simulink model "sampleModel1557"  (R2023a)
settings: Solver=VariableStepAuto  StartTime=0.0  StopTime=10.0  RelTol=1e-3
libraries: hdlsllib x3, simulink x1
settings Model: Creator=user1  LastModifiedBy=user1

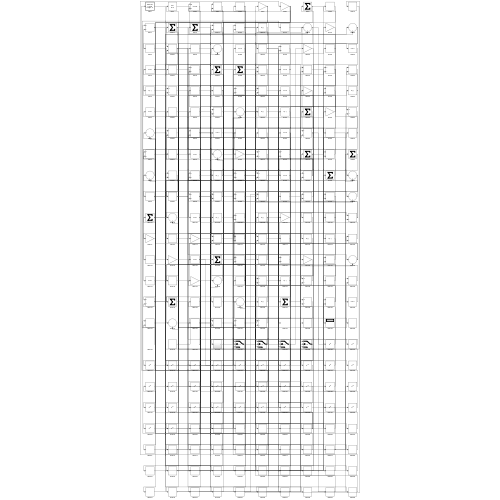
[thumbnail: Simulink's stored preview of the top-level diagram]
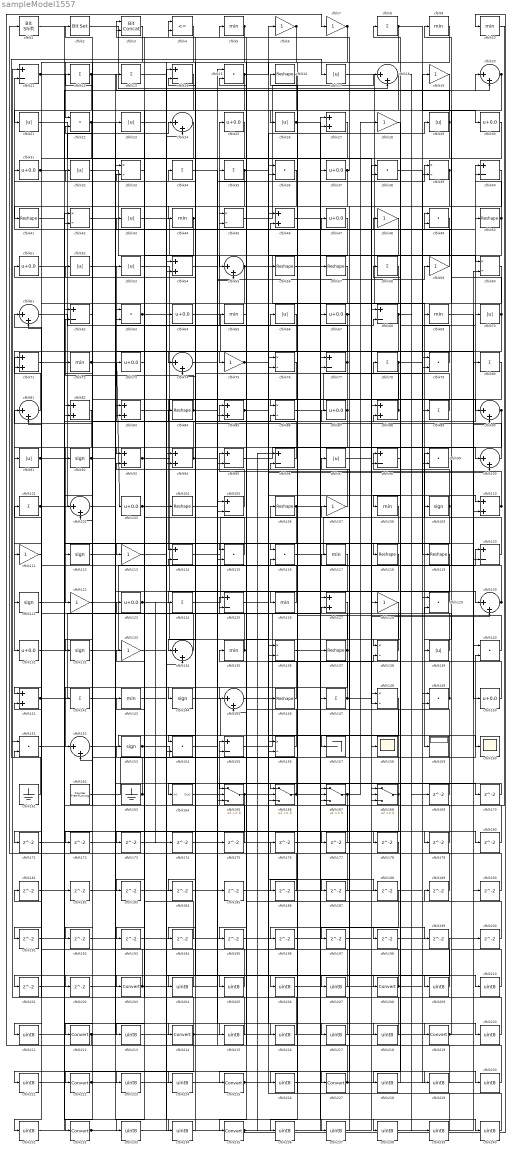
== system sampleModel1557 ==
  cfblk1 : hdlsllib/Logic and Bit Operations/Bit Shift  mode=Shift Left Logical  N=0
  cfblk{5,9..10,44,65,69,72,108,117,126,135,143} (12 alike) : MinMax
  cfblk{18,20,24,55,61,74,81,90,100,102,130,134,145,152} (14 alike) : Sum  Inputs=|++
  cfblk{8,12..13,34..35,58,78,80,89,101,124,142,147} (13 alike) : Sum  Inputs=+
  cfblk{25,30..31,37,47,51,64,67,73,87,103,123,131,150} (14 alike) : Bias  Bias=0.0  SaturateOnIntegerOverflow=off
  cfblk{16,41,50,56..57,84,104,106,118..119,137,146} (12 alike) : Reshape
  cfblk{11,14,40,62,68,77,95..96,98,105,114,120,125,155} (14 alike) : Sum  Inputs=+-
  cfblk{6..7,19,28,48,59,75,107,111,113,122,128,133} (13 alike) : Gain
  cfblk{92,109,112,121,132,144,153} (7 alike) : Signum
  cfblk{27,46,54,71,82..83,85,88,93..94,110,127,141} (13 alike) : Sum
  cfblk{15,22,36,38,49,63,79,99,115..116,129,140,149,151,154} (15 alike) : DotProduct  OutDataTypeStr=Inherit: Inherit via internal rule
  cfblk{33,39,42,45,60,76,86,136,138,148,156} (11 alike) : Product  Inputs=*/  RndMeth=Zero  SaturateOnIntegerOverflow=on
  cfblk{17,21,23,26,29,32,43,52..53,66,70,91,97,139} (14 alike) : Abs  SaturateOnIntegerOverflow=off
  cfblk157 : Terminator
  cfblk158 : Scope
  cfblk159 : Display
  cfblk160 : Scope
  cfblk161 : Ground
  cfblk162 : hdlsllib/Sources/Counter Free-Running  NumBits=16  tsamp=-1
  cfblk163 : Ground
  cfblk164 : Subsystem
      settings: LibrarySourceBlock=|
      | hdlsllib/Ports &
      | Subsystems/Subsystem
  cfblk{165..168} (4 alike) : Switch  SaturateOnIntegerOverflow=off  InputSameDT=off
  cfblk{169..202} (34 alike) : Delay  SampleTime=1
  cfblk2 : simulink/Logic and Bit Operations/Bit Set  iBit=0
      settings: LibrarySourceBlock=|
      | hdlsllib/Logic and Bit
      | Operations/Bit Set
  cfblk{203,208,212,214,219,222,225,227,232,235} (10 alike) : DataTypeConversion  SaturateOnIntegerOverflow=off  RndMeth=Floor
  cfblk{204..207,209..211,213,215..218,220..221,223..224,226,228..231,233..234,236..240} (28 alike) : DataTypeConversion  OutDataTypeStr=uint8  SaturateOnIntegerOverflow=off  RndMeth=Floor
  cfblk3 : hdlsllib/Logic and Bit Operations/Bit Concat  numInputs=2
  cfblk4 : RelationalOperator  Operator=<=  OutDataTypeStr=boolean  InputSameDT=off
  wires:
  cfblk14/1 -> cfblk232/1
  cfblk54/1 -> cfblk219/1
  cfblk67/1 -> cfblk95/2, cfblk85/2, cfblk187/1
  cfblk66/1 -> cfblk131/1
  cfblk53/1 -> cfblk126/1
  cfblk40/1 -> cfblk157/1
  cfblk19/1 -> cfblk225/1
  cfblk71/1 -> cfblk24/1
  cfblk123/1 -> cfblk146/1, cfblk174/1
  cfblk78/1 -> cfblk114/1, cfblk70/1
  cfblk95/1 -> cfblk100/1
  cfblk136/1 -> cfblk57/1
  cfblk37/1 -> cfblk4/1, cfblk44/1
  cfblk124/1 -> cfblk67/1
  cfblk146/1 -> cfblk135/1
  cfblk161/1 -> cfblk17/1
  cfblk85/1 -> cfblk145/2, cfblk188/1, cfblk220/1
  cfblk100/1 -> cfblk4/2
  cfblk111/1 -> cfblk141/1
  cfblk63/1 -> cfblk147/1, cfblk64/1
  cfblk147/1 -> cfblk16/1, cfblk130/2
  cfblk139/1 -> cfblk97/1
  cfblk87/1 -> cfblk86/1, cfblk136/2, cfblk173/1
  cfblk93/1 -> cfblk118/1, cfblk240/1
  cfblk98/1 -> cfblk8/1
  cfblk155/1 -> cfblk37/1
  cfblk156/1 -> cfblk5/1
  cfblk96/1 -> cfblk53/1
  cfblk17/1 -> cfblk159/1
  cfblk120/1 -> cfblk99/1
  cfblk56/1 -> cfblk110/1
  cfblk3/1 -> cfblk22/1
  cfblk16/1 -> cfblk113/1
  cfblk105/1 -> cfblk3/1
  cfblk112/1 -> cfblk130/1
  cfblk89/1 -> cfblk51/1
  cfblk10/1 -> cfblk155/1
  cfblk52/1 -> cfblk75/1
  cfblk9/1 -> cfblk144/1
  cfblk82/1 -> cfblk122/1
  cfblk166/1 -> cfblk32/1, cfblk81/1, cfblk120/1
  cfblk45/1 -> cfblk18/1
  cfblk114/1 -> cfblk77/2
  cfblk129/1 -> cfblk66/1
  cfblk162/1 -> cfblk140/2
  cfblk72/1 -> cfblk103/1, cfblk142/1
  cfblk61/1 -> cfblk68/2
  cfblk151/1 -> cfblk214/1
  cfblk39/1 -> cfblk171/1, cfblk228/1
  cfblk28/1 -> cfblk108/1
  cfblk118/1 -> cfblk165/1
  cfblk22/1 -> cfblk74/1, cfblk167/3, cfblk211/1
  cfblk141/1 -> cfblk56/1, cfblk180/1
  cfblk91/1 -> cfblk25/1, cfblk120/2
  cfblk2/1 -> cfblk18/2
  cfblk57/1 -> cfblk134/1
  cfblk33/1 -> cfblk203/1
  cfblk101/1 -> cfblk40/1, cfblk88/2
  cfblk55/1 -> cfblk60/1, cfblk99/2, cfblk91/1
  cfblk106/1 -> cfblk137/1, cfblk132/1
  cfblk165/1 -> cfblk138/2, cfblk223/1
  cfblk117/1 -> cfblk164/1(In1)
  cfblk25/1 -> cfblk154/1
  cfblk18/1 -> cfblk145/1, cfblk169/1
  cfblk50/1 -> cfblk40/2, cfblk148/2
  cfblk164/1(Out1) -> cfblk39/1
  cfblk21/1 -> cfblk128/1
  cfblk75/1 -> cfblk29/1, cfblk110/2
  cfblk20/1 -> cfblk69/1, cfblk26/1
  cfblk143/1 -> cfblk104/1
  cfblk79/1 -> cfblk58/1
  cfblk68/1 -> cfblk121/1, cfblk239/1
  cfblk15/1 -> cfblk6/1, cfblk152/2, cfblk100/2
  cfblk59/1 -> cfblk11/2
  cfblk130/1 -> cfblk49/1, cfblk74/2
  cfblk64/1 -> cfblk150/1
  cfblk153/1 -> cfblk155/2, cfblk116/2
  cfblk48/1 -> cfblk227/1
  cfblk7/1 -> cfblk124/1, cfblk21/1, cfblk186/1, cfblk204/1
  cfblk43/1 -> cfblk55/1
  cfblk32/1 -> cfblk79/2
  cfblk83/1 -> cfblk90/1
  cfblk133/1 -> cfblk208/1
  cfblk104/1 -> cfblk86/2
  cfblk144/1 -> cfblk167/1
  cfblk65/1 -> cfblk115/1
  cfblk167/1 -> cfblk28/1, cfblk195/1, cfblk197/1
  cfblk80/1 -> cfblk212/1
  cfblk148/1 -> cfblk156/2
  cfblk115/1 -> cfblk83/1
  cfblk74/1 -> cfblk47/1
  cfblk121/1 -> cfblk84/1
  cfblk84/1 -> cfblk62/2, cfblk49/2
  cfblk6/1 -> cfblk76/2, cfblk205/1
  cfblk132/1 -> cfblk114/2
  cfblk109/1 -> cfblk98/1, cfblk213/1
  cfblk73/1 -> cfblk93/1
  cfblk107/1 -> cfblk45/1
  cfblk138/1 -> cfblk101/1
  cfblk38/1 -> cfblk119/1
  cfblk4/1 -> cfblk41/1
  cfblk77/1 -> cfblk63/1, cfblk193/1
  cfblk24/1 -> cfblk82/2
  cfblk81/1 -> cfblk71/1
  cfblk149/1 -> cfblk125/1, cfblk85/1
  cfblk62/1 -> cfblk92/1
  cfblk69/1 -> cfblk90/2
  cfblk36/1 -> cfblk222/1
  cfblk168/1 -> cfblk117/1, cfblk226/1
  cfblk90/1 -> cfblk111/1, cfblk167/2
  cfblk102/1 -> cfblk50/1
  cfblk103/1 -> cfblk166/1, cfblk116/1
  cfblk163/1 -> cfblk83/2, cfblk72/1
  cfblk152/1 -> cfblk160/1
  cfblk70/1 -> cfblk9/1, cfblk194/1
  cfblk26/1 -> cfblk198/1, cfblk199/1
  cfblk122/1 -> cfblk89/1
  cfblk11/1 -> cfblk201/1, cfblk237/1
  cfblk47/1 -> cfblk166/2
  cfblk97/1 -> cfblk38/1
  cfblk60/1 -> cfblk102/1
  cfblk137/1 -> cfblk152/1, cfblk12/1
  cfblk140/1 -> cfblk106/1
  cfblk86/1 -> cfblk39/2
  cfblk76/1 -> cfblk105/2
  cfblk128/1 -> cfblk166/3
  cfblk150/1 -> cfblk107/1
  cfblk127/1 -> cfblk235/1
  cfblk12/1 -> cfblk73/1, cfblk81/2
  cfblk110/1 -> cfblk78/1, cfblk95/1
  cfblk8/1 -> cfblk30/1, cfblk191/1
  cfblk92/1 -> cfblk87/1, cfblk115/2
  cfblk13/1 -> cfblk154/2
  cfblk31/1 -> cfblk20/1, cfblk20/2
  cfblk99/1 -> cfblk139/1
  cfblk134/1 -> cfblk123/1
  cfblk126/1 -> cfblk61/1
  cfblk94/1 -> cfblk2/1, cfblk59/1
  cfblk44/1 -> cfblk183/1, cfblk184/1
  cfblk116/1 -> cfblk109/1
  cfblk35/1 -> cfblk112/1, cfblk179/1
  cfblk88/1 -> cfblk35/1, cfblk31/1
  cfblk135/1 -> cfblk52/1, cfblk65/1, cfblk63/2
  cfblk131/1 -> cfblk27/2
  cfblk29/1 -> cfblk13/1, cfblk138/1
  cfblk5/1 -> cfblk94/2, cfblk202/1
  cfblk169/1 -> cfblk3/2
  cfblk145/1 -> cfblk170/1
  cfblk170/1 -> cfblk165/2
  cfblk171/1 -> cfblk94/1
  cfblk58/1 -> cfblk172/1
  cfblk172/1 -> cfblk68/1
  cfblk173/1 -> cfblk55/2
  cfblk174/1 -> cfblk105/1
  cfblk154/1 -> cfblk175/1
  cfblk175/1 -> cfblk22/2
  cfblk51/1 -> cfblk177/1
  cfblk177/1 -> cfblk76/1
  cfblk119/1 -> cfblk178/1
  cfblk178/1 -> cfblk1/1
  cfblk179/1 -> cfblk102/2
  cfblk180/1 -> cfblk62/1
  cfblk181/1 -> cfblk129/1
  cfblk41/1 -> cfblk182/1
  cfblk182/1 -> cfblk156/1
  cfblk183/1 -> cfblk148/1
  cfblk184/1 -> cfblk168/2
  cfblk185/1 -> cfblk125/2
  cfblk186/1 -> cfblk141/2
  cfblk187/1 -> cfblk77/1
  cfblk189/1 -> cfblk11/1
  cfblk190/1 -> cfblk61/2
  cfblk30/1 -> cfblk192/1
  cfblk192/1 -> cfblk136/1
  cfblk193/1 -> cfblk134/2
  cfblk194/1 -> cfblk93/2
  cfblk195/1 -> cfblk88/1
  cfblk108/1 -> cfblk196/1
  cfblk196/1 -> cfblk27/1
  cfblk197/1 -> cfblk168/3
  cfblk198/1 -> cfblk60/2
  cfblk200/1 -> cfblk15/2
  cfblk201/1 -> cfblk165/3
  cfblk203/1 -> cfblk185/1, cfblk82/1
  cfblk204/1 -> cfblk33/1
  cfblk205/1 -> cfblk33/2
  cfblk176/1 -> cfblk206/1
  cfblk206/1 -> cfblk149/2
  cfblk49/1 -> cfblk207/1
  cfblk207/1 -> cfblk176/1
  cfblk208/1 -> cfblk71/2, cfblk96/2, cfblk43/1
  cfblk125/1 -> cfblk209/1
  cfblk209/1 -> cfblk133/1
  cfblk23/1 -> cfblk210/1
  cfblk210/1 -> cfblk129/2
  cfblk211/1 -> cfblk23/1
  cfblk212/1 -> cfblk7/1, cfblk24/2
  cfblk213/1 -> cfblk80/1
  cfblk214/1 -> cfblk153/1, cfblk143/1, cfblk218/1, cfblk221/1
  cfblk113/1 -> cfblk215/1
  cfblk215/1 -> cfblk151/1
  cfblk142/1 -> cfblk216/1
  cfblk216/1 -> cfblk151/2
  cfblk34/1 -> cfblk217/1
  cfblk217/1 -> cfblk181/1
  cfblk218/1 -> cfblk34/1
  cfblk219/1 -> cfblk190/1, cfblk189/1
  cfblk220/1 -> cfblk54/1
  cfblk221/1 -> cfblk54/2
  cfblk222/1 -> cfblk158/1, cfblk149/1
  cfblk223/1 -> cfblk36/1
  cfblk191/1 -> cfblk224/1
  cfblk224/1 -> cfblk36/2
  cfblk225/1 -> cfblk98/2, cfblk140/1
  cfblk226/1 -> cfblk19/1
  cfblk227/1 -> cfblk45/2, cfblk79/1
  cfblk228/1 -> cfblk48/1
  cfblk42/1 -> cfblk229/1
  cfblk229/1 -> cfblk15/1
  cfblk1/1 -> cfblk230/1
  cfblk230/1 -> cfblk42/1
  cfblk199/1 -> cfblk231/1
  cfblk231/1 -> cfblk42/2
  cfblk232/1 -> cfblk38/2, cfblk168/1
  cfblk27/1 -> cfblk233/1
  cfblk233/1 -> cfblk14/1
  cfblk202/1 -> cfblk234/1
  cfblk234/1 -> cfblk14/2
  cfblk235/1 -> cfblk10/1, cfblk96/1
  cfblk188/1 -> cfblk236/1
  cfblk236/1 -> cfblk127/1
  cfblk237/1 -> cfblk127/2
  cfblk46/1 -> cfblk238/1
  cfblk238/1 -> cfblk200/1
  cfblk239/1 -> cfblk46/1
  cfblk240/1 -> cfblk46/2

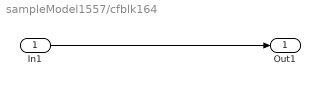
== system sampleModel1557/cfblk164 ==
  In1 : Inport
  Out1 : Outport
  wires:
  In1/1 -> Out1/1
